simulink model "eVTOL_PX4_2023b"  (R2024b)
settings: Solver=ode4  StartTime=0  StopTime=inf  FixedStep=0.01  RelTol=1e-3
values from neighbouring files (symbols this model uses):
  aDl =     [initdata.mat]
  aDr =     [initdata.mat]
  aDyn =     [initdata.mat]
  Airport = init_airport('PHNL')    [initdata_HIL_eVTOL.m]
  aLat =     [initdata.mat]
  aLon =     [initdata.mat]
  D = Prop.D    [EOM_dt_MC.m]    (also in EOM_get_alf_dt_de_prop_evtol.m = CD * QS)
  dt0 = X(2)    [EOM_get_alf_dt_de_prop_evtol.m]    (also in initdata.mat = 0.258252593971; initdata_HIL_eVTOL.m = EOM_dt_MC)
  EAS0 = TAS0 / EAS2TAS    [initdata_HIL_eVTOL.m]
  FCS = init_FCS    [initdata_HIL_eVTOL.m]
  General = init_layoutdata    [EOM_dt_MC.m]    (also in build_optimized_CA.m; initdata.mat = ; initdata_HIL_eVTOL.m)
  h0 = Con(1)    [EOM_get_alf_dt_de_prop_evtol.m]    (also in initdata.mat = 450; initdata_HIL_eVTOL.m = 50)
  mass = Con(3)    [EOM_get_alf_dt_de_prop_evtol.m]    (also in initdata.mat = 2255.54; initdata_HIL_eVTOL.m = 7)
  Motor = init_motor_evtol    [EOM_dt_MC.m]    (also in initdata.mat = []; initdata_HIL_eVTOL.m)
  Prop = init_propeller_evtol_new    [EOM_dt_MC.m]    (also in initdata_HIL_eVTOL.m)
  R2D = 180/pi    (= 57.2957795131)    [EOM_get_alf_dt_de_prop_evtol.m]    (also in init_FCS.m; init_aerodata_evtol.m; init_airport.m; initdata.mat)
  SAMPLE_TIME = 0.01    [initdata_HIL_eVTOL.m]
  theta0 = -0.0510981441662    [initdata.mat]
undefined symbols (not defined in the file or in its folder): A1, aDa, aDe, aero, asbhl20env, B1, C1, de0, Earth, Environment, INIT_Data, InitData, Kd, Kp, magnitude, Newton, pProp, Raphson, Tc, WGS84
libraries: simulink_extras x63, vrlib x48, sharedtransform x28, simulink x22, slpidlib x20, sharedutil x20, matrix_library x18, aerolibwindfilters x12, aerolibobsolete x8, aerolibasang x8, aerolibatmos2 x6, aerolibfltsims x6
(part 6 of 17)

== system eVTOL_PX4_2023b/Subsystem1/Energy & Power1/thrust_5 ==
  note: 将推力、扭矩按电机倾转角转化为向量
  note: 求桨的推力、扭矩、功率、效率
  dt : Inport
  V : Inport  Port=2
  rho : Inport  Port=3
  rpm0 : Inport  Port=4
  rpm_grid : Inport  Port=5
  i : Inport  Port=6
  Constant : Constant  Commented=on  Value=2.5
  Gain2 : Gain  Gain=-1
  Gain4 : Gain  Gain=pi/30
  Manual Switch : ManualSwitch  Commented=on  CurrentSetting=0
  Motor : Subsystem
  Mux1 : Mux  Inputs=2
  Mux2 : Mux  Inputs=3
  Mux3 : Mux  Inputs=2
  Mux4 : Mux  Inputs=3
  Product : Product  Inputs=*/
  "Propeller " : Subsystem
  Q_x : Fcn  Expr=-u[1]*cos(u[2])
  Q_y : Fcn  Expr=0
  Q_z : Fcn  Expr=u[1]*sin(u[2])
  Saturation : Saturate  UpperLimit=inf  LowerLimit=1
  T_x : Fcn  Expr=u[1]*cos(u[2])
  T_y : Fcn  Expr=0
  T_z : Fcn  Expr=-u[1]*sin(u[2])
  eta_plr : Outport  VectorParamsAs1DForOutWhenUnconnected=off
  Q : Outport  Port=2
  T : Outport  Port=3  VectorParamsAs1DForOutWhenUnconnected=off
  rpm : Outport  Port=4  VectorParamsAs1DForOutWhenUnconnected=off
  wires:
  Saturation/1 -> Motor/4(rpm0)
  rpm0/1 -> Saturation/1
  "Propeller "/2(T (N)) -> [T]
  dt/1 -> Motor/2(dt)
  Motor/1(rpm) -> rpm/1, Gain4/1, "Propeller "/1(rpm)
  "Propeller "/3(eta_p) -> eta_plr/1
  rho/1 -> [rho]
  "Propeller "/1(P_plr (w)) -> Motor/1(P_shaft), Product/1
  rpm_grid/1 -> Motor/6(rpm_grid)
  Gain4/1 -> Product/2  "omega"
  T_y/1 -> Mux2/2
  Mux1/1 -> T_z/1, T_x/1, T_y/1
  T_x/1 -> Mux2/1
  i/1 -> [i]
  T_z/1 -> Mux2/3
  Mux2/1 -> T/1
  [T] -> Mux1/1
  Mux4/1 -> Q/1
  [i] -> Mux3/2
  Q_z/1 -> Mux4/3
  Q_x/1 -> Mux4/1
  Mux3/1 -> Q_z/1, Q_x/1, Q_y/1
  Q_y/1 -> Mux4/2
  [Q] -> Mux3/1
  [i] -> Mux1/2
  Product/1 -> Gain2/1
  [V] -> Motor/3(V)
  [V] -> "Propeller "/2(V)
  [rho] -> Motor/5(rho)
  [rho] -> "Propeller "/3(rho)
  Gain2/1 -> [Q]
  Constant/1 -> Manual Switch/1
  V/1 -> [V]

== system eVTOL_PX4_2023b/Subsystem1/Energy & Power1/thrust_6 ==
  note: 将推力、扭矩按电机倾转角转化为向量
  note: 求桨的推力、扭矩、功率、效率
  dt : Inport
  V : Inport  Port=2
  rho : Inport  Port=3
  rpm0 : Inport  Port=4
  rpm_grid : Inport  Port=5
  i : Inport  Port=6
  Constant : Constant  Commented=on  Value=2.5
  Gain4 : Gain  Gain=pi/30
  Manual Switch : ManualSwitch  Commented=on  CurrentSetting=0
  Motor : Subsystem
  Mux1 : Mux  Inputs=2
  Mux2 : Mux  Inputs=3
  Mux3 : Mux  Inputs=2
  Mux4 : Mux  Inputs=3
  Product : Product  Inputs=*/
  "Propeller " : Subsystem
  Q_x : Fcn  Expr=-u[1]*cos(u[2])
  Q_y : Fcn  Expr=0
  Q_z : Fcn  Expr=u[1]*sin(u[2])
  Saturation : Saturate  UpperLimit=inf  LowerLimit=1
  T_x : Fcn  Expr=u[1]*cos(u[2])
  T_y : Fcn  Expr=0
  T_z : Fcn  Expr=-u[1]*sin(u[2])
  eta_plr : Outport  VectorParamsAs1DForOutWhenUnconnected=off
  Q : Outport  Port=2
  T : Outport  Port=3  VectorParamsAs1DForOutWhenUnconnected=off
  rpm : Outport  Port=4  VectorParamsAs1DForOutWhenUnconnected=off
  wires:
  Saturation/1 -> Motor/4(rpm0)
  rpm0/1 -> Saturation/1
  "Propeller "/2(T (N)) -> [T]
  dt/1 -> Motor/2(dt)
  Motor/1(rpm) -> rpm/1, Gain4/1, "Propeller "/1(rpm)
  "Propeller "/3(eta_p) -> eta_plr/1
  rho/1 -> [rho]
  "Propeller "/1(P_plr (w)) -> Motor/1(P_shaft), Product/1
  rpm_grid/1 -> Motor/6(rpm_grid)
  Gain4/1 -> Product/2  "omega"
  T_y/1 -> Mux2/2
  Mux1/1 -> T_z/1, T_x/1, T_y/1
  T_x/1 -> Mux2/1
  i/1 -> [i]
  T_z/1 -> Mux2/3
  Mux2/1 -> T/1
  [T] -> Mux1/1
  Mux4/1 -> Q/1
  [i] -> Mux3/2
  Q_z/1 -> Mux4/3
  Q_x/1 -> Mux4/1
  Mux3/1 -> Q_z/1, Q_x/1, Q_y/1
  Q_y/1 -> Mux4/2
  [Q] -> Mux3/1
  [i] -> Mux1/2
  [V] -> Motor/3(V)
  [V] -> "Propeller "/2(V)
  [rho] -> Motor/5(rho)
  [rho] -> "Propeller "/3(rho)
  Product/1 -> [Q]
  Constant/1 -> Manual Switch/1
  V/1 -> [V]

== system eVTOL_PX4_2023b/Subsystem1/Environment/Terrain ==
  Xe : Inport
  Terminator : Terminator
  hground_value : Constant  OutDataTypeStr=single
  hground : Outport  VectorParamsAs1DForOutWhenUnconnected=off
  wires:
  Xe/1 -> Terminator/1
  hground_value/1 -> hground/1  "hground"

== system eVTOL_PX4_2023b/Subsystem1/Environment/Wind Models ==
  Xe_x : Inport
  Ve : Inport  Port=2
  Altitude : Inport  Port=3
  DCM : Inport  Port=4
  Constant1 : Constant  Value=[0,0,0]
  Constant2 : Constant  Value=[0,0,0]
  Dot Product1 : DotProduct  OutDataTypeStr=Inherit: Inherit via internal rule
  Dot Product2 : DotProduct  OutDataTypeStr=Inherit: Inherit via internal rule
  Dryden Wind Turbulence Model (Continuous (+q -r)) : Subsystem  AncestorBlock=|  mask(Wind Turbulence Model){units=Metric (MKS), spec=MIL-F-8785C, model=Continuous Dryden (+q -r), W20=8, Wdeg=0, TurbProb=10^-4, L_high=533.4, Wingspan=7, ts=0.01, Seed=[23341 23342 23343 23344], T_on=on}
      | CustomLib_2019b/Dryden Wind Turbulence Model 
      | (Continuous (+q -r))
      mask prompts: units "aeroblks:aeroblkwind:blockWindTurbulenceModelParamUnits"; spec "aeroblks:aeroblkwind:blockWindTurbulenceModelParamSpecification"; model "aeroblks:aeroblkwind:blockWindTurbulenceModelParamModeltype"; W20 "Wind speed at 6 m defines the low-altitude intensity (m/s):"; Wdeg "Wind direction at 6 m (degrees clockwise from north):"; TurbProb "aeroblks:aeroblkwind:blockWindTurbulenceModelParamProbabilityofexceedanceofhighaltitudeintensity"; L_high "Scale length at medium/high altitudes (m):"; Wingspan "Wingspan (m):"; ts "Band limited noise sample time (sec):"; Seed "aeroblks:aeroblkwind:blockWindTurbulenceModelParamNoiseseedsugvgwgpg"; T_on "aeroblks:aeroblkwind:blockWindTurbulenceModelParamTurbulenceon"
      mask help: aeroblks:aeroblkwind:blockWindTurbulenceModelDesc
      mask init:
      | index = strfind(model,' ');
      | disp1 = model(1:index(1)-1);
      | disp2 = model(index(1)+1:index(end-1)-1);
      | disp3 = model(index(end-1)+1:end);
      | 
      | h_vec = [.5 1.75 3.75 7.5 15 25 35 45 55 65 75 80]*1000;% feet
      | sigma_vec(1,:) = [3.2 2.2 1.5 zeros(1,9)]; % ft/sec
      | sigma_vec(2,:) = [4.2 3.6 3.3 1.6 zeros(1,8)];
      | sigma_vec(3,:) = [6.6 6.9 7.4 6.7 4.6 2.7 0.4 zeros(1,5)];
      | sigma_vec(4,:) = [8.6 9.6 10.6 10.1 8.0 6.6 5.0 4.2 2.7 zeros(1,3)];
      | sigma_vec(5,:) = [11.8 13.0 16.0 15.1 11.6 9.7 8.1 8.2 7.9 4.9 3.2 2.1];
      | sigma_vec(6,:) = [15.6 17.6 23.0 23.6 22.1 20.0 16.0 15.1 12.1 7.9 6.2 5.1];
      | sigma_vec(7,:) = [18.7 21.5 28.4 30.2 30.7 31.0 25.2 23.1 17.5 10.7 8.4 7.2];
      | max_height_low = 1000;
      | if strcmp(spec,'MIL-F-8785C')
      |     min_height_high = 2000;
      | else
      | 	min_height_high = 1750;
      | end
      | [ports] = aeroicon('aeroblkwindturb2','icon');
      | 
      | dt=ts;
      settings: LibrarySourceBlock=|
      | CustomLib_2019b/Dryden Wind Turbulence Model
      | (Continuous (+q -r))
      mask Help: eval('asbhelp(''Dryden Wind Turbulence Model (Continuous)'')');
      mask TypeOptions units: aeroblks:aeroblkwind:blockWindTurbulenceModelParamComboMetricMKS | aeroblks:aeroblkwind:blockWindTurbulenceModelParamComboEnglishVelocityinfts | aeroblks:aeroblkwind:blockWindTurbulenceModelParamComboEnglishVelocityinkts
      mask TypeOptions spec: aeroblks:aeroblkwind:blockWindTurbulenceModelParamComboMILF8785C | aeroblks:aeroblkwind:blockWindTurbulenceModelParamComboMILHDBK1797 | aeroblks:aeroblkwind:blockWindTurbulenceModelParamComboMILHDBK1797B
      mask TypeOptions model: aeroblks:aeroblkwind:blockWindTurbulenceModelParamComboContinuousVonKarmanqr1 | aeroblks:aeroblkwind:blockWindTurbulenceModelParamComboContinuousVonKarmanqr2 | aeroblks:aeroblkwind:blockWindTurbulenceModelParamComboContinuousVonKarmanqr3 | aeroblks:aeroblkwind:blockWindTurbulenceModelParamComboContinuousDrydenqr1 | aeroblks:aeroblkwind:blockWindTurbulenceModelParamComboContinuousDrydenqr2 | aeroblks:aeroblkwind:blockWindTurbulenceModelParamComboContinuousDrydenqr3 | aeroblks:aeroblkwind:blockWindTurbulenceModelParamComboDiscreteDrydenqr1 | aeroblks:aeroblkwind:blockWindTurbulenceModelParamComboDiscreteDrydenqr2 | aeroblks:aeroblkwind:blockWindTurbulenceModelParamComboDiscreteDrydenqr3
      mask Callback model: aeroicon('aeroblkwindturb2');
      mask TypeOptions TurbProb: aeroblks:aeroblkwind:blockWindTurbulenceModelParamCombo2x101 | aeroblks:aeroblkwind:blockWindTurbulenceModelParamCombo101 | aeroblks:aeroblkwind:blockWindTurbulenceModelParamCombo102Light | aeroblks:aeroblkwind:blockWindTurbulenceModelParamCombo103Moderate | aeroblks:aeroblkwind:blockWindTurbulenceModelParamCombo104 | aeroblks:aeroblkwind:blockWindTurbulenceModelParamCombo105Severe | aeroblks:aeroblkwind:blockWindTurbulenceModelParamCombo106
      mask DialogControl units Prompt: Units:
      mask DialogControl spec Prompt: Specification:
      mask DialogControl model Prompt: Model type:
      mask DialogControl TurbProb Prompt: Probability of exceedance of high-altitude intensity:
      mask DialogControl Seed Prompt: Noise seeds [ug vg wg pg]:
      mask DialogControl T_on Prompt: Turbulence on
      mask Display:
      | port_label(ports(1).type,ports(1).port,ports(1).txt,'texmode','on');
      | port_label(ports(2).type,ports(2).port,ports(2).txt,'texmode','on');
      | port_label(ports(3).type,ports(3).port,ports(3).txt,'texmode','on');
      | port_label(ports(4).type,ports(4).port,ports(4).txt,'texmode','on');
      | port_label(ports(5).type,ports(5).port,ports(5).txt,'texmode','on');
  Gain4 : Gain  Gain=[1,1,1]
  Manual Switch1 : ManualSwitch  CurrentSetting=0
  Manual Switch2 : ManualSwitch  CurrentSetting=0
  Sqrt : Sqrt
  vt1 : Math  Operator=sqrt  SignedPower=on
  wind scp2 : Scope
  wind_mag scp : Scope
  windangular scp : Scope
  windspeed scp : Scope
  ug,vg,wg1 : Outport  VectorParamsAs1DForOutWhenUnconnected=off
  pg,qg,rg1 : Outport  Port=2  VectorParamsAs1DForOutWhenUnconnected=off
  wires:
  Manual Switch2/1 -> ug,vg,wg1/1  "WindVelocity"
  Dryden Wind Turbulence Model (Continuous (+q -r))/1(ug,vg,wg) -> Gain4/1, windspeed scp/1, Dot Product2/2, Dot Product2/1  "Vw"
  Dryden Wind Turbulence Model (Continuous (+q -r))/2(pg,qg,rg) -> Manual Switch1/1, windangular scp/1  "WindAngularRates"
  Constant1/1 -> Manual Switch1/2
  Altitude/1 -> [Altitude]
  vt1/1 -> [Airspeed]  "Airspeed"
  Constant2/1 -> Manual Switch2/2
  [Airspeed] -> Dryden Wind Turbulence Model (Continuous (+q -r))/2(Airspeed)  "Airspeed"
  DCM/1 -> [DCM]
  Ve/1 -> Dot Product1/2, Dot Product1/1
  Manual Switch1/1 -> pg,qg,rg1/1  "WindAngularRates"
  Gain4/1 -> Manual Switch2/1  "WindVelocity"
  [Altitude] -> Dryden Wind Turbulence Model (Continuous (+q -r))/1(Altitude)
  Dot Product2/1 -> Sqrt/1
  [DCM] -> Dryden Wind Turbulence Model (Continuous (+q -r))/3(DCM)
  Dot Product1/1 -> vt1/1
  Sqrt/1 -> wind_mag scp/1  "wind_mag"
  Xe_x/1 -> [x]
  [x] -> wind scp2/1

== system eVTOL_PX4_2023b/Subsystem1/Environment1/Terrain ==
  Xe : Inport
  Terminator : Terminator
  hground_value : Constant  OutDataTypeStr=single
  hground : Outport  VectorParamsAs1DForOutWhenUnconnected=off
  wires:
  Xe/1 -> Terminator/1
  hground_value/1 -> hground/1  "hground"

== system eVTOL_PX4_2023b/Subsystem1/Environment1/Wind Models ==
  Xe_x : Inport
  Ve : Inport  Port=2
  Altitude : Inport  Port=3
  DCM : Inport  Port=4
  Constant1 : Constant  Value=[0,0,0]
  Constant2 : Constant  Value=[0,0,0]
  Dot Product1 : DotProduct  OutDataTypeStr=Inherit: Inherit via internal rule
  Dot Product2 : DotProduct  OutDataTypeStr=Inherit: Inherit via internal rule
  Dryden Wind Turbulence Model (Continuous (+q -r)) : Subsystem  AncestorBlock=|  mask(Wind Turbulence Model){units=Metric (MKS), spec=MIL-F-8785C, model=Continuous Dryden (+q -r), W20=8, Wdeg=0, TurbProb=10^-4, L_high=533.4, Wingspan=7, ts=0.01, Seed=[23341 23342 23343 23344], T_on=on}
      | CustomLib_2019b/Dryden Wind Turbulence Model 
      | (Continuous (+q -r))
      mask prompts: units "aeroblks:aeroblkwind:blockWindTurbulenceModelParamUnits"; spec "aeroblks:aeroblkwind:blockWindTurbulenceModelParamSpecification"; model "aeroblks:aeroblkwind:blockWindTurbulenceModelParamModeltype"; W20 "Wind speed at 6 m defines the low-altitude intensity (m/s):"; Wdeg "Wind direction at 6 m (degrees clockwise from north):"; TurbProb "aeroblks:aeroblkwind:blockWindTurbulenceModelParamProbabilityofexceedanceofhighaltitudeintensity"; L_high "Scale length at medium/high altitudes (m):"; Wingspan "Wingspan (m):"; ts "Band limited noise sample time (sec):"; Seed "aeroblks:aeroblkwind:blockWindTurbulenceModelParamNoiseseedsugvgwgpg"; T_on "aeroblks:aeroblkwind:blockWindTurbulenceModelParamTurbulenceon"
      mask help: aeroblks:aeroblkwind:blockWindTurbulenceModelDesc
      mask init: same as eVTOL_PX4_2023b/Subsystem1/Environment/Wind Models/Dryden Wind Turbulence Model (Continuous (+q -r))
      settings: LibrarySourceBlock=|
      | CustomLib_2019b/Dryden Wind Turbulence Model
      | (Continuous (+q -r))
      mask Help: eval('asbhelp(''Dryden Wind Turbulence Model (Continuous)'')');
      mask TypeOptions units: aeroblks:aeroblkwind:blockWindTurbulenceModelParamComboMetricMKS | aeroblks:aeroblkwind:blockWindTurbulenceModelParamComboEnglishVelocityinfts | aeroblks:aeroblkwind:blockWindTurbulenceModelParamComboEnglishVelocityinkts
      mask TypeOptions spec: aeroblks:aeroblkwind:blockWindTurbulenceModelParamComboMILF8785C | aeroblks:aeroblkwind:blockWindTurbulenceModelParamComboMILHDBK1797 | aeroblks:aeroblkwind:blockWindTurbulenceModelParamComboMILHDBK1797B
      mask TypeOptions model: aeroblks:aeroblkwind:blockWindTurbulenceModelParamComboContinuousVonKarmanqr1 | aeroblks:aeroblkwind:blockWindTurbulenceModelParamComboContinuousVonKarmanqr2 | aeroblks:aeroblkwind:blockWindTurbulenceModelParamComboContinuousVonKarmanqr3 | aeroblks:aeroblkwind:blockWindTurbulenceModelParamComboContinuousDrydenqr1 | aeroblks:aeroblkwind:blockWindTurbulenceModelParamComboContinuousDrydenqr2 | aeroblks:aeroblkwind:blockWindTurbulenceModelParamComboContinuousDrydenqr3 | aeroblks:aeroblkwind:blockWindTurbulenceModelParamComboDiscreteDrydenqr1 | aeroblks:aeroblkwind:blockWindTurbulenceModelParamComboDiscreteDrydenqr2 | aeroblks:aeroblkwind:blockWindTurbulenceModelParamComboDiscreteDrydenqr3
      mask Callback model: aeroicon('aeroblkwindturb2');
      mask TypeOptions TurbProb: aeroblks:aeroblkwind:blockWindTurbulenceModelParamCombo2x101 | aeroblks:aeroblkwind:blockWindTurbulenceModelParamCombo101 | aeroblks:aeroblkwind:blockWindTurbulenceModelParamCombo102Light | aeroblks:aeroblkwind:blockWindTurbulenceModelParamCombo103Moderate | aeroblks:aeroblkwind:blockWindTurbulenceModelParamCombo104 | aeroblks:aeroblkwind:blockWindTurbulenceModelParamCombo105Severe | aeroblks:aeroblkwind:blockWindTurbulenceModelParamCombo106
      mask DialogControl units Prompt: Units:
      mask DialogControl spec Prompt: Specification:
      mask DialogControl model Prompt: Model type:
      mask DialogControl TurbProb Prompt: Probability of exceedance of high-altitude intensity:
      mask DialogControl Seed Prompt: Noise seeds [ug vg wg pg]:
      mask DialogControl T_on Prompt: Turbulence on
      mask Display:
      | port_label(ports(1).type,ports(1).port,ports(1).txt,'texmode','on');
      | port_label(ports(2).type,ports(2).port,ports(2).txt,'texmode','on');
      | port_label(ports(3).type,ports(3).port,ports(3).txt,'texmode','on');
      | port_label(ports(4).type,ports(4).port,ports(4).txt,'texmode','on');
      | port_label(ports(5).type,ports(5).port,ports(5).txt,'texmode','on');
  Gain4 : Gain  Gain=[1,1,1]
  Manual Switch1 : ManualSwitch  CurrentSetting=0
  Manual Switch2 : ManualSwitch  CurrentSetting=0
  Sqrt : Sqrt
  vt1 : Math  Operator=sqrt  SignedPower=on
  wind scp2 : Scope
  wind_mag scp : Scope
  windangular scp : Scope
  windspeed scp : Scope
  ug,vg,wg1 : Outport  VectorParamsAs1DForOutWhenUnconnected=off
  pg,qg,rg1 : Outport  Port=2  VectorParamsAs1DForOutWhenUnconnected=off
  wires:
  Manual Switch2/1 -> ug,vg,wg1/1  "WindVelocity"
  Dryden Wind Turbulence Model (Continuous (+q -r))/1(ug,vg,wg) -> Gain4/1, windspeed scp/1, Dot Product2/2, Dot Product2/1  "Vw"
  Dryden Wind Turbulence Model (Continuous (+q -r))/2(pg,qg,rg) -> Manual Switch1/1, windangular scp/1  "WindAngularRates"
  Constant1/1 -> Manual Switch1/2
  Altitude/1 -> [Altitude]
  vt1/1 -> [Airspeed]  "Airspeed"
  Constant2/1 -> Manual Switch2/2
  [Airspeed] -> Dryden Wind Turbulence Model (Continuous (+q -r))/2(Airspeed)  "Airspeed"
  DCM/1 -> [DCM]
  Ve/1 -> Dot Product1/2, Dot Product1/1
  Manual Switch1/1 -> pg,qg,rg1/1  "WindAngularRates"
  Gain4/1 -> Manual Switch2/1  "WindVelocity"
  [Altitude] -> Dryden Wind Turbulence Model (Continuous (+q -r))/1(Altitude)
  Dot Product2/1 -> Sqrt/1
  [DCM] -> Dryden Wind Turbulence Model (Continuous (+q -r))/3(DCM)
  Dot Product1/1 -> vt1/1
  Sqrt/1 -> wind_mag scp/1  "wind_mag"
  Xe_x/1 -> [x]
  [x] -> wind scp2/1

== system eVTOL_PX4_2023b/Subsystem1/airframe/Flight Conditions ==
  EnvmData : Inport
  PlantData : Inport  Port=2
  Bus Selector1 : BusSelector  OutputSignals=WindVelocity,a,AirDensity,WindAngularRates,Po,To,g
  Bus Selector2 : BusSelector  OutputSignals=Xe,Ve,Vb,pqr,DCM_be
  Constant1 : Constant  Value=Airport.Elevation_m
  Constant2 : Constant  Value=1.225
  Demux : Demux  Outputs=2
  Derivative : Derivative  CoefficientInTFapproximation=100
  Divide : Product  Inputs=*/
  Divide1 : Product  Inputs=**
  Dynamic Pressure : aerolibasang/Dynamic Pressure
  Flat Earth to LLA1 : aerolibtransform2/Flat Earth to LLA  units=Metric (MKS)  ptype=Earth (WGS84)  F=1/298.257223563  R=6378137  refPosPort=off  LL0=InitData.LLA(1:2)*R2D  psi=0
  "Incidence, Sideslip, & Airspeed" : Subsystem  AncestorBlock=aerolibasang/Incidence, Sideslip, & Airspeed  mask(Incidence,Sideslip,&Airspeed){}
      mask help: Calculate the angles between the body and the velocity vector (incidence and sideslip), and the velocity magnitude from the components in body axes (Vb).
      settings: LibrarySourceBlock=|
      | aerolibasang/Incidence, Sideslip,
      | & Airspeed
      mask Help: web(asbhelp('incidence'));
      mask Display:
      | port_label('input',1,'V_b','texmode','on');
      | port_label('output',1,'\alpha','texmode','on');
      | port_label('output',2,'\beta','texmode','on');
      | port_label('output',3,'V','texmode','on');
  Mach Number : aerolibasang/Mach Number
  Product : Product  Multiplication=Matrix(*)
  Product1 : Product  Multiplication=Matrix(*)
  Sqrt : Sqrt
  Subsystem : Subsystem
  Sum1 : Sum  Inputs=+-|  InputSameDT=on  SaturateOnIntegerOverflow=on  OutDataTypeStr=Inherit: Same as first input
  Sum2 : Sum  Inputs=|+-  InputSameDT=on  SaturateOnIntegerOverflow=on  OutDataTypeStr=Inherit: Same as first input
  Terminator : Terminator
  Vw_b : Scope
  Vw_e : Scope
  lat_deg : Outport  VectorParamsAs1DForOutWhenUnconnected=off
  lon_deg : Outport  Port=2  VectorParamsAs1DForOutWhenUnconnected=off
  amsl : Outport  Port=3  VectorParamsAs1DForOutWhenUnconnected=off
  Alpha : Outport  Port=4  VectorParamsAs1DForOutWhenUnconnected=off
  AlphaDot : Outport  Port=5  VectorParamsAs1DForOutWhenUnconnected=off
  Beta : Outport  Port=6  VectorParamsAs1DForOutWhenUnconnected=off
  V : Outport  Port=7  VectorParamsAs1DForOutWhenUnconnected=off
  EAS : Outport  Port=8  VectorParamsAs1DForOutWhenUnconnected=off
  pqrWind : Outport  Port=9  VectorParamsAs1DForOutWhenUnconnected=off
  Mach : Outport  Port=10  VectorParamsAs1DForOutWhenUnconnected=off
  Qbar : Outport  Port=11  InitialOutput=0  VectorParamsAs1DForOutWhenUnconnected=off
  gamma : Outport  Port=12  InitialOutput=0  VectorParamsAs1DForOutWhenUnconnected=off
  chi : Outport  Port=13  InitialOutput=0  VectorParamsAs1DForOutWhenUnconnected=off
  Po : Outport  Port=14  VectorParamsAs1DForOutWhenUnconnected=off
  To : Outport  Port=15  VectorParamsAs1DForOutWhenUnconnected=off
  g : Outport  Port=16  VectorParamsAs1DForOutWhenUnconnected=off
  wires:
  Derivative/1 -> AlphaDot/1
  Bus Selector1/4 -> Product1/2  "<WindAngularRates>"
  Subsystem/1(gamma) -> gamma/1
  PlantData/1 -> Bus Selector2/1
  Sum2/1 -> "Incidence, Sideslip, & Airspeed"/1(Vb), Mach Number/1, Dynamic Pressure/1  "VA(b)"
  Subsystem/2(chi) -> chi/1
  Bus Selector2/3 -> Sum2/1  "<Vb>"
  Subsystem/3(V) -> Terminator/1
  Product1/1 -> Sum1/2
  Bus Selector1/5 -> Po/1  "<Po>"
  Mach Number/1 -> Mach/1  "Mach"
  "Incidence, Sideslip, & Airspeed"/1(Alpha) -> Alpha/1, Derivative/1  "Alpha"
  Product/1 -> Vw_b/1, Sum2/2
  Bus Selector2/2 -> Subsystem/1(<Ve>)  "<Ve>"
  "Incidence, Sideslip, & Airspeed"/2(Beta) -> Beta/1  "Beta"
  Dynamic Pressure/1 -> Qbar/1  "qbar"
  Bus Selector1/2 -> Mach Number/2  "<a>"
  Bus Selector2/5 -> Product/1, Product1/1  "<DCM_be>"
  Bus Selector2/4 -> Sum1/1  "<pqr>"
  Sum1/1 -> pqrWind/1
  EnvmData/1 -> Bus Selector1/1
  Bus Selector1/3 -> Divide/1, Dynamic Pressure/2  "<AirDensity>"
  Bus Selector1/1 -> Product/2, Vw_e/1  "<WindVelocity>"
  Bus Selector1/7 -> g/1  "<g>"
  Bus Selector1/6 -> To/1  "<To>"
  Demux/1 -> lat_deg/1  "lat_deg"
  Demux/2 -> lon_deg/1  "lon_deg"
  Flat Earth to LLA1/2 -> amsl/1  "amsl"
  Flat Earth to LLA1/1 -> Demux/1
  Constant1/1 -> Flat Earth to LLA1/2
  Bus Selector2/1 -> Flat Earth to LLA1/1  "<Xe>"
  Constant2/1 -> Divide/2
  Divide1/1 -> EAS/1
  Divide/1 -> Sqrt/1
  "Incidence, Sideslip, & Airspeed"/3(V) -> Divide1/1, V/1  "V"
  Sqrt/1 -> Divide1/2

== system eVTOL_PX4_2023b/Subsystem1/airframe/force moment ==
  note: force and moment in body fixed axis coordination
  PlantData : Inport
  Act_surface : Inport  Port=2
  prop : Inport  Port=3
  EnvmData : Inport  Port=4
  Add : Sum  Inputs=++++
  Add1 : Sum  Inputs=++++
  Disturbance : Constant  Value=[0,10,0]
  Disturbance1 : Constant  Value=[0,0,0]
  F_Gear_in_b scp : Scope
  F_tot : Scope
  Gear&FM in body axis : Subsystem
  Gear&FM in body axis1 : Subsystem  Commented=on
  M_Gear scp : Scope
  M_tot : Scope
  Manual Switch : ManualSwitch  CurrentSetting=0
  Motor moment scp : Scope
  Scope{2..4,6} (4 alike) : Scope
  Thrust&M in body axis : Subsystem
  aero F&M in body axis : Subsystem
  gravity in body axis : Subsystem
  Fb (X Y Z) : Outport  VectorParamsAs1DForOutWhenUnconnected=off
  M (L M N) : Outport  Port=2  VectorParamsAs1DForOutWhenUnconnected=off
  wires:
  Thrust&M in body axis/1(f_T) -> Add/1, Scope4/1
  gravity in body axis/1(Fb) -> Add/3, Scope3/1
  Thrust&M in body axis/2(m_T) -> Add1/1, Motor moment scp/1
  aero F&M in body axis/2(M (L M N)) -> Scope6/1, Add1/2
  Add1/1 -> M_tot/1, M (L M N)/1
  Add/1 -> F_tot/1, Fb (X Y Z)/1
  PlantData/1 -> aero F&M in body axis/1(PlantData), Gear&FM in body axis/1(PlantData), gravity in body axis/1(PlantData)
  Act_surface/1 -> aero F&M in body axis/2(Act_surface)
  EnvmData/1 -> gravity in body axis/2(EnvmData)
  Gear&FM in body axis/1(F_Gear) -> Add/4, F_Gear_in_b scp/1
  Gear&FM in body axis/2(M_Gear) -> Add1/3, M_Gear scp/1
  aero F&M in body axis/1(Fb (X Y Z)) -> Add/2, Scope2/1
  Disturbance/1 -> Manual Switch/1
  Manual Switch/1 -> Add1/4
  Disturbance1/1 -> Manual Switch/2
  prop/1 -> Thrust&M in body axis/1(prop)

== system eVTOL_PX4_2023b/Subsystem1/airframe1/Flight Conditions ==
  EnvmData : Inport
  PlantData : Inport  Port=2
  Bus Selector1 : BusSelector  OutputSignals=WindVelocity,a,AirDensity,WindAngularRates,Po,To,g
  Bus Selector2 : BusSelector  OutputSignals=Ve,Vb,pqr,DCM_be,Xe
  Constant1 : Constant  Value=Airport.Elevation_m
  Constant2 : Constant  Value=1.225
  Demux : Demux  Outputs=2
  Derivative : Derivative  CoefficientInTFapproximation=100
  Divide : Product  Inputs=*/
  Divide1 : Product  Inputs=**
  Dynamic Pressure : aerolibasang/Dynamic Pressure
  Flat Earth to LLA1 : aerolibtransform2/Flat Earth to LLA  units=Metric (MKS)  ptype=Earth (WGS84)  F=1/298.257223563  R=6378137  refPosPort=off  LL0=InitData.LLA(1:2)*R2D  psi=0
  "Incidence, Sideslip, & Airspeed" : Subsystem  AncestorBlock=aerolibasang/Incidence, Sideslip, & Airspeed  mask(Incidence,Sideslip,&Airspeed){}
      mask help: Calculate the angles between the body and the velocity vector (incidence and sideslip), and the velocity magnitude from the components in body axes (Vb).
      settings: LibrarySourceBlock=|
      | aerolibasang/Incidence, Sideslip,
      | & Airspeed
      mask Help: web(asbhelp('incidence'));
      mask Display:
      | port_label('input',1,'V_b','texmode','on');
      | port_label('output',1,'\alpha','texmode','on');
      | port_label('output',2,'\beta','texmode','on');
      | port_label('output',3,'V','texmode','on');
  Mach Number : aerolibasang/Mach Number
  Product : Product  Multiplication=Matrix(*)
  Product1 : Product  Multiplication=Matrix(*)
  Sqrt : Sqrt
  Subsystem : Subsystem
  Sum1 : Sum  Inputs=+-|  InputSameDT=on  SaturateOnIntegerOverflow=on  OutDataTypeStr=Inherit: Same as first input
  Sum2 : Sum  Inputs=|+-  InputSameDT=on  SaturateOnIntegerOverflow=on  OutDataTypeStr=Inherit: Same as first input
  Terminator : Terminator
  Va_b : Scope
  Vk_b : Scope
  Vw_b : Scope
  Vw_e : Scope
  Alpha : Outport  VectorParamsAs1DForOutWhenUnconnected=off
  AlphaDot : Outport  Port=2  VectorParamsAs1DForOutWhenUnconnected=off
  Beta : Outport  Port=3  VectorParamsAs1DForOutWhenUnconnected=off
  V : Outport  Port=4  VectorParamsAs1DForOutWhenUnconnected=off
  pqrWind : Outport  Port=5  VectorParamsAs1DForOutWhenUnconnected=off
  Mach : Outport  Port=6  VectorParamsAs1DForOutWhenUnconnected=off
  Qbar : Outport  Port=7  InitialOutput=0  VectorParamsAs1DForOutWhenUnconnected=off
  gamma : Outport  Port=8  InitialOutput=0  VectorParamsAs1DForOutWhenUnconnected=off
  chi : Outport  Port=9  InitialOutput=0  VectorParamsAs1DForOutWhenUnconnected=off
  Po : Outport  Port=10  VectorParamsAs1DForOutWhenUnconnected=off
  To : Outport  Port=11  VectorParamsAs1DForOutWhenUnconnected=off
  g : Outport  Port=12  VectorParamsAs1DForOutWhenUnconnected=off
  lat_deg : Outport  Port=13  VectorParamsAs1DForOutWhenUnconnected=off
  lon_deg : Outport  Port=14  VectorParamsAs1DForOutWhenUnconnected=off
  amsl : Outport  Port=15  VectorParamsAs1DForOutWhenUnconnected=off
  EAS : Outport  Port=16  VectorParamsAs1DForOutWhenUnconnected=off
  wires:
  Derivative/1 -> AlphaDot/1
  Bus Selector1/4 -> Product1/2  "<WindAngularRates>"
  Subsystem/1(gamma) -> gamma/1
  PlantData/1 -> Bus Selector2/1
  Sum2/1 -> "Incidence, Sideslip, & Airspeed"/1(Vb), Va_b/1, Mach Number/1, Dynamic Pressure/1  "VA(b)"
  Subsystem/2(chi) -> chi/1
  Bus Selector2/2 -> Sum2/1, Vk_b/1  "<Vb>"
  Subsystem/3(V) -> Terminator/1
  Product1/1 -> Sum1/2
  Bus Selector1/5 -> Po/1  "<Po>"
  Mach Number/1 -> Mach/1  "Mach"
  "Incidence, Sideslip, & Airspeed"/1(Alpha) -> Derivative/1, Alpha/1  "Alpha"
  Product/1 -> Vw_b/1, Sum2/2
  Bus Selector2/1 -> Subsystem/1(<Ve>)  "<Ve>"
  "Incidence, Sideslip, & Airspeed"/2(Beta) -> Beta/1  "Beta"
  Dynamic Pressure/1 -> Qbar/1  "qbar"
  Bus Selector1/2 -> Mach Number/2  "<a>"
  Bus Selector2/4 -> Product/1, Product1/1  "<DCM_be>"
  Bus Selector2/3 -> Sum1/1  "<pqr>"
  Sum1/1 -> pqrWind/1
  EnvmData/1 -> Bus Selector1/1
  Bus Selector1/1 -> Product/2, Vw_e/1  "<WindVelocity>"
  Bus Selector1/7 -> g/1  "<g>"
  Bus Selector1/6 -> To/1  "<To>"
  Flat Earth to LLA1/1 -> Demux/1
  Flat Earth to LLA1/2 -> amsl/1  "amsl"
  Constant1/1 -> Flat Earth to LLA1/2
  Demux/1 -> lat_deg/1  "lat_deg"
  Demux/2 -> lon_deg/1  "lon_deg"
  Bus Selector2/5 -> Flat Earth to LLA1/1  "<Xe>"
  Divide/1 -> Sqrt/1
  Bus Selector1/3 -> Divide/1, Dynamic Pressure/2  "<AirDensity>"
  Constant2/1 -> Divide/2
  Divide1/1 -> EAS/1
  Sqrt/1 -> Divide1/2
  "Incidence, Sideslip, & Airspeed"/3(V) -> Divide1/1, V/1  "V"

== system eVTOL_PX4_2023b/Subsystem1/airframe1/force moment ==
  note: force and moment in body fixed axis coordination
  PlantData : Inport
  Act_surface : Inport  Port=2
  prop : Inport  Port=3
  EnvmData : Inport  Port=4
  Add : Sum  Inputs=++++
  Add1 : Sum  Inputs=++++
  Disturbance : Constant  Value=[0,10,0]
  Disturbance1 : Constant  Value=[0,0,0]
  F_Gear_in_b scp : Scope  Commented=on
  F_Gear_in_b scp1 : Scope
  Gear&FM in body axis : Subsystem  Commented=on
  Gear&FM in body axis1 : Subsystem
  M_Gear scp : Scope  Commented=on
  M_Gear scp1 : Scope
  Manual Switch : ManualSwitch  CurrentSetting=0
  Motor moment scp : Scope
  Scope{,1..4,6} (6 alike) : Scope
  Thrust&M in body axis : Subsystem
  aero F&M in body axis : Subsystem
  gravity in body axis : Subsystem
  Fb (X Y Z) : Outport  VectorParamsAs1DForOutWhenUnconnected=off
  M (L M N) : Outport  Port=2  VectorParamsAs1DForOutWhenUnconnected=off
  wires:
  Thrust&M in body axis/1(f_T) -> Add/1, Scope4/1
  gravity in body axis/1(Fb) -> Add/3, Scope3/1
  Thrust&M in body axis/2(m_T) -> Add1/1, Motor moment scp/1
  aero F&M in body axis/2(M (L M N)) -> Scope6/1, Add1/2
  Add1/1 -> Scope1/1, M (L M N)/1
  Add/1 -> Scope/1, Fb (X Y Z)/1
  Act_surface/1 -> aero F&M in body axis/2(Act_surface)
  EnvmData/1 -> gravity in body axis/2(EnvmData)
  Gear&FM in body axis/1(F_Gear) -> F_Gear_in_b scp/1
  Gear&FM in body axis/2(M_Gear) -> M_Gear scp/1
  aero F&M in body axis/1(Fb (X Y Z)) -> Add/2, Scope2/1
  Disturbance/1 -> Manual Switch/1
  Manual Switch/1 -> Add1/4
  Disturbance1/1 -> Manual Switch/2
  prop/1 -> Thrust&M in body axis/1(prop)
  PlantData/1 -> Gear&FM in body axis1/1(PlantData), aero F&M in body axis/1(PlantData), gravity in body axis/1(PlantData)
  Gear&FM in body axis1/2(M_Gear) -> Add1/3, M_Gear scp1/1
  Gear&FM in body axis1/1(F_Gear) -> F_Gear_in_b scp1/1, Add/4

== system eVTOL_PX4_2023b/Subsystem2/Energy & Power/V_prop1 ==
  note: 将速度矢量投影到桨轴
  pqr : Inport
  pos : Inport  Port=2
  i : Inport  Port=3
  Vb : Inport  Port=4
  Cross Product4 : matrix_library/Cross Product
  Display1 : Display
  Display2 : Display
  Display8 : Display
  Sum2 : Sum  Inputs=|++
  v_b to v_prop : Subsystem
  V : Outport
  wires:
  pos/1 -> Cross Product4/2
  pqr/1 -> Cross Product4/1
  Vb/1 -> Display2/1, Sum2/2
  i/1 -> v_b to v_prop/2(i)
  Cross Product4/1 -> Display8/1, Sum2/1
  Sum2/1 -> Display1/1, v_b to v_prop/1(V_body)
  v_b to v_prop/1(V) -> V/1

== system eVTOL_PX4_2023b/Subsystem2/Energy & Power/V_prop2 ==
  note: 将速度矢量投影到桨轴
  pqr : Inport
  pos : Inport  Port=2
  i : Inport  Port=3
  Vb : Inport  Port=4
  Cross Product4 : matrix_library/Cross Product
  Sum2 : Sum  Inputs=|++
  v_b to v_prop : Subsystem
  V : Outport
  wires:
  pos/1 -> Cross Product4/2
  pqr/1 -> Cross Product4/1
  Vb/1 -> Sum2/2
  i/1 -> v_b to v_prop/2(i)
  Cross Product4/1 -> Sum2/1
  Sum2/1 -> v_b to v_prop/1(V_body)
  v_b to v_prop/1(V) -> V/1

== system eVTOL_PX4_2023b/Subsystem2/Energy & Power/V_prop3 ==
  note: 将速度矢量投影到桨轴
  pqr : Inport
  pos : Inport  Port=2
  i : Inport  Port=3
  Va : Inport  Port=4
  Cross Product4 : matrix_library/Cross Product
  Sum2 : Sum  Inputs=|++
  v_b to v_prop : Subsystem
  V : Outport
  wires:
  pos/1 -> Cross Product4/2
  pqr/1 -> Cross Product4/1
  Va/1 -> Sum2/2
  i/1 -> v_b to v_prop/2(i)
  Cross Product4/1 -> Sum2/1
  Sum2/1 -> v_b to v_prop/1(V_body)
  v_b to v_prop/1(V) -> V/1

== system eVTOL_PX4_2023b/Subsystem2/Energy & Power/V_prop4 ==
  note: 将速度矢量投影到桨轴
  pqr : Inport
  pos : Inport  Port=2
  i : Inport  Port=3
  Va : Inport  Port=4
  Cross Product4 : matrix_library/Cross Product
  Sum2 : Sum  Inputs=|++
  v_b to v_prop : Subsystem
  V : Outport
  wires:
  pos/1 -> Cross Product4/2
  pqr/1 -> Cross Product4/1
  Va/1 -> Sum2/2
  i/1 -> v_b to v_prop/2(i)
  Cross Product4/1 -> Sum2/1
  Sum2/1 -> v_b to v_prop/1(V_body)
  v_b to v_prop/1(V) -> V/1

== system eVTOL_PX4_2023b/Subsystem2/Energy & Power/V_prop5 ==
  note: 将速度矢量投影到桨轴
  pqr : Inport
  pos : Inport  Port=2
  i : Inport  Port=3
  Va : Inport  Port=4
  Cross Product4 : matrix_library/Cross Product
  Sum2 : Sum  Inputs=|++
  v_b to v_prop : Subsystem
  V : Outport
  wires:
  pos/1 -> Cross Product4/2
  pqr/1 -> Cross Product4/1
  Va/1 -> Sum2/2
  i/1 -> v_b to v_prop/2(i)
  Cross Product4/1 -> Sum2/1
  Sum2/1 -> v_b to v_prop/1(V_body)
  v_b to v_prop/1(V) -> V/1

== system eVTOL_PX4_2023b/Subsystem2/Energy & Power/V_prop6 ==
  note: 将速度矢量投影到桨轴
  pqr : Inport
  pos : Inport  Port=2
  i : Inport  Port=3
  Va : Inport  Port=4
  Cross Product4 : matrix_library/Cross Product
  Sum2 : Sum  Inputs=|++
  v_b to v_prop : Subsystem
  V : Outport
  wires:
  pos/1 -> Cross Product4/2
  pqr/1 -> Cross Product4/1
  Va/1 -> Sum2/2
  i/1 -> v_b to v_prop/2(i)
  Cross Product4/1 -> Sum2/1
  Sum2/1 -> v_b to v_prop/1(V_body)
  v_b to v_prop/1(V) -> V/1

== system eVTOL_PX4_2023b/Subsystem2/Energy & Power/thrust_1 ==
  note: 将推力、扭矩按电机倾转角转化为向量
  note: 求桨的推力、扭矩、功率、效率
  dt : Inport
  V : Inport  Port=2
  rho : Inport  Port=3
  rpm0 : Inport  Port=4
  theta_b : Inport  Port=5
  i : Inport  Port=6
  Constant : Constant  Commented=on  Value=2.5
  Gain2 : Gain  Gain=-1
  Gain4 : Gain  Gain=pi/30
  Manual Switch : ManualSwitch  Commented=on  CurrentSetting=0
  Motor : Subsystem
  Mux1 : Mux  Inputs=2
  Mux2 : Mux  Inputs=3
  Mux3 : Mux  Inputs=2
  Mux4 : Mux  Inputs=3
  Product : Product  Inputs=*/
  "Propeller " : Subsystem
  Q_x : Fcn  Expr=-u[1]*cos(u[2])
  Q_y : Fcn  Expr=0
  Q_z : Fcn  Expr=u[1]*sin(u[2])
  Saturation : Saturate  UpperLimit=inf  LowerLimit=1
  T_x : Fcn  Expr=u[1]*cos(u[2])
  T_y : Fcn  Expr=0
  T_z : Fcn  Expr=-u[1]*sin(u[2])
  eta_plr : Outport  VectorParamsAs1DForOutWhenUnconnected=off
  Q : Outport  Port=2
  T : Outport  Port=3  VectorParamsAs1DForOutWhenUnconnected=off
  rpm : Outport  Port=4  VectorParamsAs1DForOutWhenUnconnected=off
  wires:
  Saturation/1 -> Motor/4(rpm0)
  rpm0/1 -> Saturation/1
  "Propeller "/2(T (N)) -> [T]
  dt/1 -> Motor/2(dt)
  Motor/1(rpm) -> rpm/1, Gain4/1, "Propeller "/1(rpm)
  "Propeller "/3(eta_p) -> eta_plr/1
  rho/1 -> [rho]
  "Propeller "/1(P_plr (w)) -> Motor/1(P_shaft), Product/1
  theta_b/1 -> Motor/6(theta_b), "Propeller "/4(theta_b)
  Gain4/1 -> Product/2  "omega"
  Product/1 -> Gain2/1
  T_y/1 -> Mux2/2
  Mux1/1 -> T_z/1, T_x/1, T_y/1
  T_x/1 -> Mux2/1
  i/1 -> [i]
  T_z/1 -> Mux2/3
  Mux2/1 -> T/1
  [T] -> Mux1/1
  Mux4/1 -> Q/1
  [i] -> Mux3/2
  Q_z/1 -> Mux4/3
  Q_x/1 -> Mux4/1
  Mux3/1 -> Q_z/1, Q_x/1, Q_y/1
  Q_y/1 -> Mux4/2
  [Q] -> Mux3/1
  [i] -> Mux1/2
  Gain2/1 -> [Q]
  [V] -> Motor/3(V)
  [V] -> "Propeller "/2(V)
  [rho] -> Motor/5(rho)
  [rho] -> "Propeller "/3(rho)
  Constant/1 -> Manual Switch/1
  V/1 -> [V]

== system eVTOL_PX4_2023b/Subsystem2/Energy & Power/thrust_2 ==
  note: 将推力、扭矩按电机倾转角转化为向量
  note: 求桨的推力、扭矩、功率、效率
  dt : Inport
  V : Inport  Port=2
  rho : Inport  Port=3
  rpm0 : Inport  Port=4
  theta_b : Inport  Port=5
  i : Inport  Port=6
  Constant : Constant  Commented=on  Value=2.5
  Gain4 : Gain  Gain=pi/30
  Manual Switch : ManualSwitch  Commented=on  CurrentSetting=0
  Motor : Subsystem
  Mux1 : Mux  Inputs=2
  Mux2 : Mux  Inputs=3
  Mux3 : Mux  Inputs=2
  Mux4 : Mux  Inputs=3
  Product : Product  Inputs=*/
  "Propeller " : Subsystem
  Q_x : Fcn  Expr=-u[1]*cos(u[2])
  Q_y : Fcn  Expr=0
  Q_z : Fcn  Expr=u[1]*sin(u[2])
  Saturation : Saturate  UpperLimit=inf  LowerLimit=1
  T_x : Fcn  Expr=u[1]*cos(u[2])
  T_y : Fcn  Expr=0
  T_z : Fcn  Expr=-u[1]*sin(u[2])
  eta_plr : Outport  VectorParamsAs1DForOutWhenUnconnected=off
  Q : Outport  Port=2
  T : Outport  Port=3  VectorParamsAs1DForOutWhenUnconnected=off
  rpm : Outport  Port=4  VectorParamsAs1DForOutWhenUnconnected=off
  wires:
  Saturation/1 -> Motor/4(rpm0)
  rpm0/1 -> Saturation/1
  "Propeller "/2(T (N)) -> [T]
  dt/1 -> Motor/2(dt)
  Motor/1(rpm) -> rpm/1, Gain4/1, "Propeller "/1(rpm)
  "Propeller "/3(eta_p) -> eta_plr/1
  rho/1 -> [rho]
  "Propeller "/1(P_plr (w)) -> Motor/1(P_shaft), Product/1
  theta_b/1 -> Motor/6(theta_b), "Propeller "/4(theta_b)
  Gain4/1 -> Product/2  "omega"
  T_y/1 -> Mux2/2
  Mux1/1 -> T_z/1, T_x/1, T_y/1
  T_x/1 -> Mux2/1
  i/1 -> [i]
  T_z/1 -> Mux2/3
  Mux2/1 -> T/1
  [T] -> Mux1/1
  Mux4/1 -> Q/1
  [i] -> Mux3/2
  Q_z/1 -> Mux4/3
  Q_x/1 -> Mux4/1
  Mux3/1 -> Q_z/1, Q_x/1, Q_y/1
  Q_y/1 -> Mux4/2
  [Q] -> Mux3/1
  [i] -> Mux1/2
  Product/1 -> [Q]
  [V] -> Motor/3(V)
  [V] -> "Propeller "/2(V)
  [rho] -> Motor/5(rho)
  [rho] -> "Propeller "/3(rho)
  Constant/1 -> Manual Switch/1
  V/1 -> [V]

== system eVTOL_PX4_2023b/Subsystem2/Energy & Power/thrust_3 ==
  note: 将推力、扭矩按电机倾转角转化为向量
  note: 求桨的推力、扭矩、功率、效率
  dt : Inport
  V : Inport  Port=2
  rho : Inport  Port=3
  rpm0 : Inport  Port=4
  theta_b : Inport  Port=5
  i : Inport  Port=6
  Constant : Constant  Commented=on  Value=2.5
  Gain4 : Gain  Gain=pi/30
  Manual Switch : ManualSwitch  Commented=on  CurrentSetting=0
  Motor : Subsystem
  Mux1 : Mux  Inputs=2
  Mux2 : Mux  Inputs=3
  Mux3 : Mux  Inputs=2
  Mux4 : Mux  Inputs=3
  Product : Product  Inputs=*/
  "Propeller " : Subsystem
  Q_x : Fcn  Expr=-u[1]*cos(u[2])
  Q_y : Fcn  Expr=0
  Q_z : Fcn  Expr=u[1]*sin(u[2])
  Saturation : Saturate  UpperLimit=inf  LowerLimit=1
  T_x : Fcn  Expr=u[1]*cos(u[2])
  T_y : Fcn  Expr=0
  T_z : Fcn  Expr=-u[1]*sin(u[2])
  eta_plr : Outport  VectorParamsAs1DForOutWhenUnconnected=off
  Q : Outport  Port=2
  T : Outport  Port=3  VectorParamsAs1DForOutWhenUnconnected=off
  rpm : Outport  Port=4  VectorParamsAs1DForOutWhenUnconnected=off
  wires:
  Saturation/1 -> Motor/4(rpm0)
  rpm0/1 -> Saturation/1
  "Propeller "/2(T (N)) -> [T]
  dt/1 -> Motor/2(dt)
  Motor/1(rpm) -> rpm/1, Gain4/1, "Propeller "/1(rpm)
  "Propeller "/3(eta_p) -> eta_plr/1
  rho/1 -> [rho]
  "Propeller "/1(P_plr (w)) -> Motor/1(P_shaft), Product/1
  theta_b/1 -> Motor/6(theta_b), "Propeller "/4(theta_b)
  Gain4/1 -> Product/2  "omega"
  T_y/1 -> Mux2/2
  Mux1/1 -> T_z/1, T_x/1, T_y/1
  T_x/1 -> Mux2/1
  i/1 -> [i]
  T_z/1 -> Mux2/3
  Mux2/1 -> T/1
  [T] -> Mux1/1
  Mux4/1 -> Q/1
  [i] -> Mux3/2
  Q_z/1 -> Mux4/3
  Q_x/1 -> Mux4/1
  Mux3/1 -> Q_z/1, Q_x/1, Q_y/1
  Q_y/1 -> Mux4/2
  [Q] -> Mux3/1
  [i] -> Mux1/2
  Product/1 -> [Q]
  [V] -> Motor/3(V)
  [V] -> "Propeller "/2(V)
  [rho] -> Motor/5(rho)
  [rho] -> "Propeller "/3(rho)
  Constant/1 -> Manual Switch/1
  V/1 -> [V]

== system eVTOL_PX4_2023b/Subsystem2/Energy & Power/thrust_4 ==
  note: 将推力、扭矩按电机倾转角转化为向量
  note: 求桨的推力、扭矩、功率、效率
  dt : Inport
  V : Inport  Port=2
  rho : Inport  Port=3
  rpm0 : Inport  Port=4
  theta_b : Inport  Port=5
  i : Inport  Port=6
  Constant : Constant  Commented=on  Value=2.5
  Gain2 : Gain  Gain=-1
  Gain4 : Gain  Gain=pi/30
  Manual Switch : ManualSwitch  Commented=on  CurrentSetting=0
  Motor : Subsystem
  Mux1 : Mux  Inputs=2
  Mux2 : Mux  Inputs=3
  Mux3 : Mux  Inputs=2
  Mux4 : Mux  Inputs=3
  Product : Product  Inputs=*/
  "Propeller " : Subsystem
  Q_x : Fcn  Expr=-u[1]*cos(u[2])
  Q_y : Fcn  Expr=0
  Q_z : Fcn  Expr=u[1]*sin(u[2])
  Saturation : Saturate  UpperLimit=inf  LowerLimit=1
  T_x : Fcn  Expr=u[1]*cos(u[2])
  T_y : Fcn  Expr=0
  T_z : Fcn  Expr=-u[1]*sin(u[2])
  eta_plr : Outport  VectorParamsAs1DForOutWhenUnconnected=off
  Q : Outport  Port=2
  T : Outport  Port=3  VectorParamsAs1DForOutWhenUnconnected=off
  rpm : Outport  Port=4  VectorParamsAs1DForOutWhenUnconnected=off
  wires:
  Saturation/1 -> Motor/4(rpm0)
  rpm0/1 -> Saturation/1
  "Propeller "/2(T (N)) -> [T]
  dt/1 -> Motor/2(dt)
  Motor/1(rpm) -> rpm/1, Gain4/1, "Propeller "/1(rpm)
  "Propeller "/3(eta_p) -> eta_plr/1
  rho/1 -> [rho]
  "Propeller "/1(P_plr (w)) -> Motor/1(P_shaft), Product/1
  theta_b/1 -> Motor/6(theta_b), "Propeller "/4(theta_b)
  Gain4/1 -> Product/2  "omega"
  T_y/1 -> Mux2/2
  Mux1/1 -> T_z/1, T_x/1, T_y/1
  T_x/1 -> Mux2/1
  i/1 -> [i]
  T_z/1 -> Mux2/3
  Mux2/1 -> T/1
  [T] -> Mux1/1
  Mux4/1 -> Q/1
  [i] -> Mux3/2
  Q_z/1 -> Mux4/3
  Q_x/1 -> Mux4/1
  Mux3/1 -> Q_z/1, Q_x/1, Q_y/1
  Q_y/1 -> Mux4/2
  [Q] -> Mux3/1
  [i] -> Mux1/2
  Product/1 -> Gain2/1
  [V] -> Motor/3(V)
  [V] -> "Propeller "/2(V)
  [rho] -> Motor/5(rho)
  [rho] -> "Propeller "/3(rho)
  Gain2/1 -> [Q]
  Constant/1 -> Manual Switch/1
  V/1 -> [V]

== system eVTOL_PX4_2023b/Subsystem2/Energy & Power/thrust_5 ==
  note: 将推力、扭矩按电机倾转角转化为向量
  note: 求桨的推力、扭矩、功率、效率
  dt : Inport
  V : Inport  Port=2
  rho : Inport  Port=3
  rpm0 : Inport  Port=4
  theta_b : Inport  Port=5
  i : Inport  Port=6
  Constant : Constant  Commented=on  Value=2.5
  Gain2 : Gain  Gain=-1
  Gain4 : Gain  Gain=pi/30
  Manual Switch : ManualSwitch  Commented=on  CurrentSetting=0
  Motor : Subsystem
  Mux1 : Mux  Inputs=2
  Mux2 : Mux  Inputs=3
  Mux3 : Mux  Inputs=2
  Mux4 : Mux  Inputs=3
  Product : Product  Inputs=*/
  "Propeller " : Subsystem
  Q_x : Fcn  Expr=-u[1]*cos(u[2])
  Q_y : Fcn  Expr=0
  Q_z : Fcn  Expr=u[1]*sin(u[2])
  Saturation : Saturate  UpperLimit=inf  LowerLimit=1
  T_x : Fcn  Expr=u[1]*cos(u[2])
  T_y : Fcn  Expr=0
  T_z : Fcn  Expr=-u[1]*sin(u[2])
  eta_plr : Outport  VectorParamsAs1DForOutWhenUnconnected=off
  Q : Outport  Port=2
  T : Outport  Port=3  VectorParamsAs1DForOutWhenUnconnected=off
  rpm : Outport  Port=4  VectorParamsAs1DForOutWhenUnconnected=off
  wires:
  Saturation/1 -> Motor/4(rpm0)
  rpm0/1 -> Saturation/1
  "Propeller "/2(T (N)) -> [T]
  dt/1 -> Motor/2(dt)
  Motor/1(rpm) -> rpm/1, Gain4/1, "Propeller "/1(rpm)
  "Propeller "/3(eta_p) -> eta_plr/1
  rho/1 -> [rho]
  "Propeller "/1(P_plr (w)) -> Motor/1(P_shaft), Product/1
  theta_b/1 -> Motor/6(theta_b), "Propeller "/4(theta_b)
  Gain4/1 -> Product/2  "omega"
  T_y/1 -> Mux2/2
  Mux1/1 -> T_z/1, T_x/1, T_y/1
  T_x/1 -> Mux2/1
  i/1 -> [i]
  T_z/1 -> Mux2/3
  Mux2/1 -> T/1
  [T] -> Mux1/1
  Mux4/1 -> Q/1
  [i] -> Mux3/2
  Q_z/1 -> Mux4/3
  Q_x/1 -> Mux4/1
  Mux3/1 -> Q_z/1, Q_x/1, Q_y/1
  Q_y/1 -> Mux4/2
  [Q] -> Mux3/1
  [i] -> Mux1/2
  Product/1 -> Gain2/1
  [V] -> Motor/3(V)
  [V] -> "Propeller "/2(V)
  [rho] -> Motor/5(rho)
  [rho] -> "Propeller "/3(rho)
  Gain2/1 -> [Q]
  Constant/1 -> Manual Switch/1
  V/1 -> [V]

== system eVTOL_PX4_2023b/Subsystem2/Energy & Power/thrust_6 ==
  note: 将推力、扭矩按电机倾转角转化为向量
  note: 求桨的推力、扭矩、功率、效率
  dt : Inport
  V : Inport  Port=2
  rho : Inport  Port=3
  rpm0 : Inport  Port=4
  theta_b : Inport  Port=5
  i : Inport  Port=6
  Constant : Constant  Commented=on  Value=2.5
  Gain4 : Gain  Gain=pi/30
  Manual Switch : ManualSwitch  Commented=on  CurrentSetting=0
  Motor : Subsystem
  Mux1 : Mux  Inputs=2
  Mux2 : Mux  Inputs=3
  Mux3 : Mux  Inputs=2
  Mux4 : Mux  Inputs=3
  Product : Product  Inputs=*/
  "Propeller " : Subsystem
  Q_x : Fcn  Expr=-u[1]*cos(u[2])
  Q_y : Fcn  Expr=0
  Q_z : Fcn  Expr=u[1]*sin(u[2])
  Saturation : Saturate  UpperLimit=inf  LowerLimit=1
  T_x : Fcn  Expr=u[1]*cos(u[2])
  T_y : Fcn  Expr=0
  T_z : Fcn  Expr=-u[1]*sin(u[2])
  eta_plr : Outport  VectorParamsAs1DForOutWhenUnconnected=off
  Q : Outport  Port=2
  T : Outport  Port=3  VectorParamsAs1DForOutWhenUnconnected=off
  rpm : Outport  Port=4  VectorParamsAs1DForOutWhenUnconnected=off
  wires:
  Saturation/1 -> Motor/4(rpm0)
  rpm0/1 -> Saturation/1
  "Propeller "/2(T (N)) -> [T]
  dt/1 -> Motor/2(dt)
  Motor/1(rpm) -> rpm/1, Gain4/1, "Propeller "/1(rpm)
  "Propeller "/3(eta_p) -> eta_plr/1
  rho/1 -> [rho]
  "Propeller "/1(P_plr (w)) -> Motor/1(P_shaft), Product/1
  theta_b/1 -> Motor/6(theta_b), "Propeller "/4(theta_b)
  Gain4/1 -> Product/2  "omega"
  T_y/1 -> Mux2/2
  Mux1/1 -> T_z/1, T_x/1, T_y/1
  T_x/1 -> Mux2/1
  i/1 -> [i]
  T_z/1 -> Mux2/3
  Mux2/1 -> T/1
  [T] -> Mux1/1
  Mux4/1 -> Q/1
  [i] -> Mux3/2
  Q_z/1 -> Mux4/3
  Q_x/1 -> Mux4/1
  Mux3/1 -> Q_z/1, Q_x/1, Q_y/1
  Q_y/1 -> Mux4/2
  [Q] -> Mux3/1
  [i] -> Mux1/2
  [V] -> Motor/3(V)
  [V] -> "Propeller "/2(V)
  [rho] -> Motor/5(rho)
  [rho] -> "Propeller "/3(rho)
  Product/1 -> [Q]
  Constant/1 -> Manual Switch/1
  V/1 -> [V]

== system eVTOL_PX4_2023b/Subsystem2/Environment/Terrain ==
  Xe : Inport
  Terminator : Terminator
  hground_value : Constant  OutDataTypeStr=single
  hground : Outport  VectorParamsAs1DForOutWhenUnconnected=off
  wires:
  Xe/1 -> Terminator/1
  hground_value/1 -> hground/1  "hground"
